simulink model "Turntable_close"  (R2017b)
settings: Solver=FixedStepAuto  StartTime=0.0  StopTime=10  FixedStep=0.0005  RelTol=1e-3
values from neighbouring files (symbols this model uses):
  bClose = 1    [sweep.m]
  bFt = 1    [sweep.m]
  bTf = 0    [sweep.m]
  fre = fre_array(i)    [sweep.m]
  J = 1.076    [sweep.m]
  Kps = 1.077250780790937e+02    (= 107.725078079)    [sweep.m]
  Kt = 24.812626200641272    (= 24.8126262006)    [sweep.m]
  Kv = 0.12    [sweep.m]
  L = 0.733240176511722    (= 0.733240176512)    [sweep.m]
  mag = 10 .^ (turntable_bode.mag / 20)    [sweep.m]    (also in test.m = ET205(1: 75, 1))
  r = 80.116666666666666667    (= 80.1166666667)    [sweep.m]
  t_off = 10    [sweep.m]
  Type = 1    [sweep.m]
settings Model: Creator=Vera  LastModifiedBy=surunbing
settings OptimizationCC: LifeSpan=inf
settings DebuggingCC: SFExecutionAtInitializationDiag=none
settings CodeAppCC: StateflowObjectComments=on

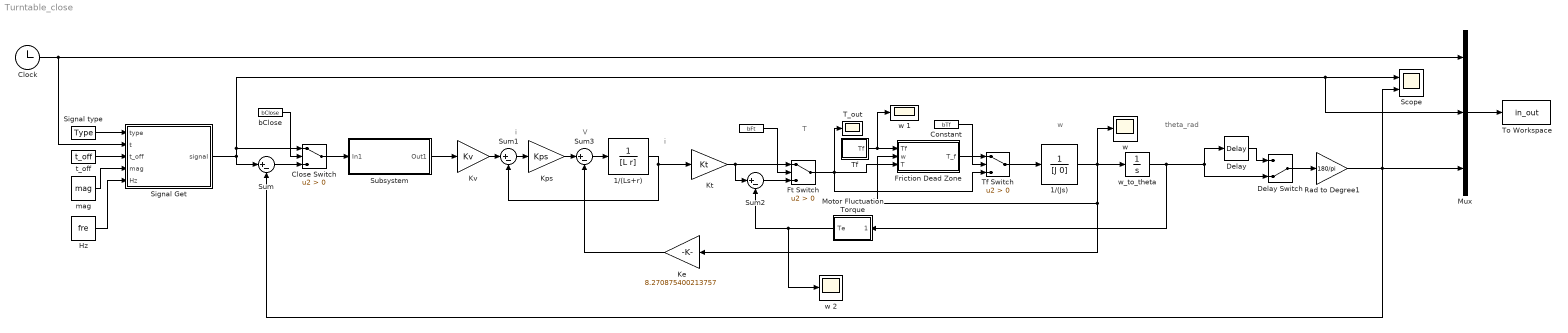
== system Turntable_close ==
  note: i
  note: w
  note: V
  note: i
  note: T
  note: theta_rad
  " " : Constant  Value=bFt
  " Delay Switch" : ManualSwitch  CurrentSetting=0
  " bClose" : Constant  Value=bClose
  1/(Js) : TransferFcn  Denominator=[J 0]
  1/(Ls+r) : TransferFcn  Denominator=[L r]
  Clock : Clock
  Close Switch : Switch  Criteria=u2 > Threshold
  Constant : Constant  Value=bTf
  Delay : TransportDelay  DelayTime=0.003763900000000
  Friction Dead Zone : MATLAB Function  TreatAsAtomicUnit=on
  Ft Switch : Switch  Criteria=u2 > Threshold
  Hz : Constant  Value=fre
  Ke : Gain  Gain=8.270875400213757
  Kps : Gain  Gain=Kps
  Kt : Gain  Gain=Kt
  Kv : Gain  Gain=Kv
  Motor Fluctuation Torque : Subsystem
  Mux : Mux  Inputs=3
  Rad to Degree1 : Gain  Gain=180/pi
  Scope : Scope  NumInputPorts=2
  Signal Get : MATLAB Function  TreatAsAtomicUnit=on
  Signal type : Constant  Value=Type
  Subsystem : Subsystem
  Sum{,1..3} (4 alike) : Sum  Inputs=|+-
  T_out : Scope
  Tf : Subsystem
  Tf Switch : Switch  Criteria=u2 > Threshold
  To Workspace : ToWorkspace  VariableName=in_out  SampleTime=-1
  mag : Constant  Value=mag
  t_off : Constant  Value=t_off
  "w " : Scope
  w 1 : Scope
  w 2 : Scope
  w_to_theta : Integrator
  wires:
  t_off/1 -> Signal Get/3(t_off)
  Clock/1 -> Mux/1, Signal Get/2(t)
  mag/1 -> Signal Get/4(mag)
  Hz/1 -> Signal Get/5(Hz)
  Kv/1 -> Sum1/1
  Motor Fluctuation Torque/1(Te) -> w 2/1, Sum2/2
  Tf/1(Tf) -> w 1/1, Friction Dead Zone/1(Tf)
  1/(Ls+r)/1 -> Sum1/2, Kt/1
  Rad to Degree1/1 -> Sum/2, Scope/2, Mux/3
  Sum3/1 -> 1/(Ls+r)/1
  Delay/1 -> " Delay Switch"/1
  w_to_theta/1 -> Delay/1, " Delay Switch"/2, Motor Fluctuation Torque/1(theta)
  " Delay Switch"/1 -> Rad to Degree1/1
  1/(Js)/1 -> "w "/1, w_to_theta/1, Friction Dead Zone/2(w), Ke/1
  Ke/1 -> Sum3/2
  Sum1/1 -> Kps/1
  Kt/1 -> Ft Switch/1, Sum2/1
  Kps/1 -> Sum3/1
  Mux/1 -> To Workspace/1
  Signal type/1 -> Signal Get/1(type)
  Subsystem/1(Out1) -> Kv/1
  Signal Get/1(signal) -> Sum/1, Close Switch/1, Mux/2, Scope/1
  Tf Switch/1 -> 1/(Js)/1
  Friction Dead Zone/1(T_f) -> Tf Switch/1
  Constant/1 -> Tf Switch/2
  Sum2/1 -> Ft Switch/3
  " "/1 -> Ft Switch/2
  Ft Switch/1 -> Friction Dead Zone/3(T), Tf Switch/3, T_out/1
  Close Switch/1 -> Subsystem/1(In1)
  Sum/1 -> Close Switch/3
  " bClose"/1 -> Close Switch/2

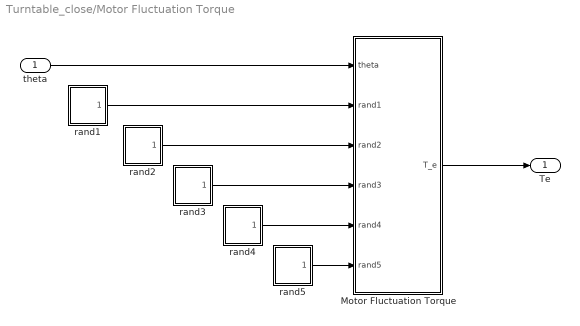
== system Turntable_close/Motor Fluctuation Torque ==
  theta : Inport
  Motor Fluctuation Torque : MATLAB Function  TreatAsAtomicUnit=on
  rand1 : Subsystem
  rand2 : Subsystem
  rand3 : Subsystem
  rand4 : Subsystem
  rand5 : Subsystem
  Te : Outport
  wires:
  theta/1 -> Motor Fluctuation Torque/1(theta)
  rand1/1(rand1) -> Motor Fluctuation Torque/2(rand1)
  rand2/1(rand2) -> Motor Fluctuation Torque/3(rand2)
  rand3/1(rand3) -> Motor Fluctuation Torque/4(rand3)
  rand4/1(rand4) -> Motor Fluctuation Torque/5(rand4)
  rand5/1(rand5) -> Motor Fluctuation Torque/6(rand5)
  Motor Fluctuation Torque/1(T_e) -> Te/1

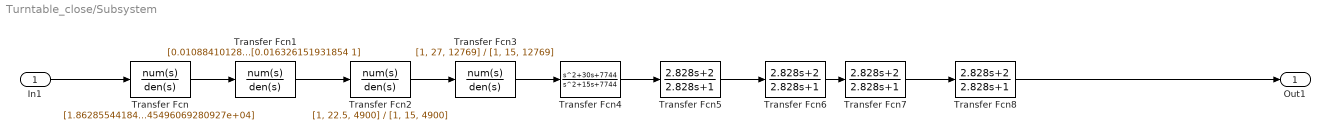
== system Turntable_close/Subsystem ==
  In1 : Inport
  Transfer Fcn : TransferFcn  Numerator=[1.862855441845868e+03, 4.791184320340544e+05, 4.845577407565945e+05]  Denominator=[0.069518879142540, 1.156462324547402e+02, 6.745496069280927e+04]
  Transfer Fcn1 : TransferFcn  Numerator=[0.010884101287903, 1] * 0.633290558182777  Denominator=[0.016326151931854 1]
  Transfer Fcn2 : TransferFcn  Numerator=[1, 22.5, 4900]  Denominator=[1, 15, 4900]
  Transfer Fcn3 : TransferFcn  Numerator=[1, 27, 12769]  Denominator=[1, 15, 12769]
  Transfer Fcn4 : TransferFcn  Numerator=[1, 30, 7744]  Denominator=[1, 15, 7744]
  Transfer Fcn{5..8} (4 alike) : TransferFcn  Numerator=[2.828, 2]  Denominator=[2.828, 1]
  Out1 : Outport
  wires:
  In1/1 -> Transfer Fcn/1
  Transfer Fcn/1 -> Transfer Fcn1/1
  Transfer Fcn1/1 -> Transfer Fcn2/1
  Transfer Fcn2/1 -> Transfer Fcn3/1
  Transfer Fcn3/1 -> Transfer Fcn4/1
  Transfer Fcn4/1 -> Transfer Fcn5/1
  Transfer Fcn5/1 -> Transfer Fcn6/1
  Transfer Fcn6/1 -> Transfer Fcn7/1
  Transfer Fcn7/1 -> Transfer Fcn8/1
  Transfer Fcn8/1 -> Out1/1

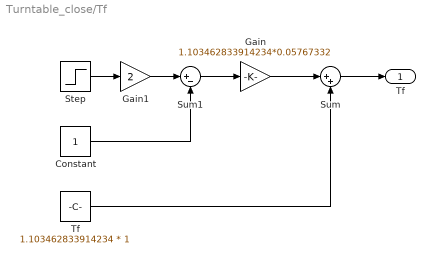
== system Turntable_close/Tf ==
  Constant : Constant
  Gain : Gain  Gain=1.103462833914234*0.05767332
  Gain1 : Gain  Gain=2
  Step : Step  Time=0  After=rand  SampleTime=0
  Sum : Sum  Inputs=|++
  Sum1 : Sum  Inputs=|+-
  "Tf " : Constant  Value=1.103462833914234 * 1  VectorParams1D=off
  Tf : Outport
  wires:
  Gain/1 -> Sum/1
  "Tf "/1 -> Sum/2
  Sum/1 -> Tf/1
  Step/1 -> Gain1/1
  Gain1/1 -> Sum1/1
  Constant/1 -> Sum1/2
  Sum1/1 -> Gain/1

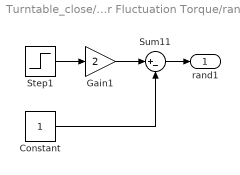
== system Turntable_close/Motor Fluctuation Torque/rand1 ==
  Constant : Constant
  Gain1 : Gain  Gain=2
  Step1 : Step  Time=0  After=rand  SampleTime=0
  Sum11 : Sum  Inputs=|+-
  rand1 : Outport
  wires:
  Step1/1 -> Gain1/1
  Gain1/1 -> Sum11/1
  Constant/1 -> Sum11/2
  Sum11/1 -> rand1/1

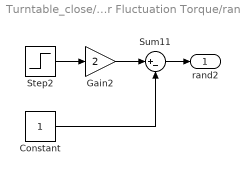
== system Turntable_close/Motor Fluctuation Torque/rand2 ==
  Constant : Constant
  Gain2 : Gain  Gain=2
  Step2 : Step  Time=0  After=rand  SampleTime=0
  Sum11 : Sum  Inputs=|+-
  rand2 : Outport
  wires:
  Step2/1 -> Gain2/1
  Gain2/1 -> Sum11/1
  Constant/1 -> Sum11/2
  Sum11/1 -> rand2/1

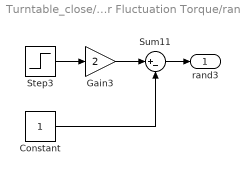
== system Turntable_close/Motor Fluctuation Torque/rand3 ==
  Constant : Constant
  Gain3 : Gain  Gain=2
  Step3 : Step  Time=0  After=rand  SampleTime=0
  Sum11 : Sum  Inputs=|+-
  rand3 : Outport
  wires:
  Sum11/1 -> rand3/1
  Constant/1 -> Sum11/2
  Gain3/1 -> Sum11/1
  Step3/1 -> Gain3/1

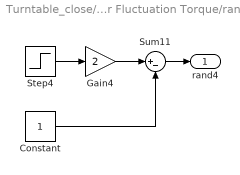
== system Turntable_close/Motor Fluctuation Torque/rand4 ==
  Constant : Constant
  Gain4 : Gain  Gain=2
  Step4 : Step  Time=0  After=rand  SampleTime=0
  Sum11 : Sum  Inputs=|+-
  rand4 : Outport
  wires:
  Step4/1 -> Gain4/1
  Gain4/1 -> Sum11/1
  Constant/1 -> Sum11/2
  Sum11/1 -> rand4/1

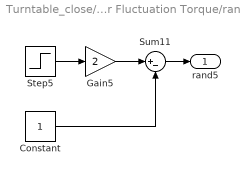
== system Turntable_close/Motor Fluctuation Torque/rand5 ==
  Constant : Constant
  Gain5 : Gain  Gain=2
  Step5 : Step  Time=0  After=rand  SampleTime=0
  Sum11 : Sum  Inputs=|+-
  rand5 : Outport
  wires:
  Sum11/1 -> rand5/1
  Constant/1 -> Sum11/2
  Gain5/1 -> Sum11/1
  Step5/1 -> Gain5/1

== matlab function Turntable_close/Signal Get ==
  data: type input; t input; t_off input; mag input; signal output; Hz input
function signal = fcn(type, t, t_off, mag, Hz)
signal = 0;
switch type
    case 1
        w = 2 * pi * Hz;
        if((t >= 0) && (t < 1))
            signal = t * mag * sin(w * t);
        elseif((t >= 1) && (t < t_off - 1))
            signal = mag * sin(w * t);
        elseif((t >= (t_off - 1)) && (t < t_off))
            signal = -mag * (t - t_off) * sin(w * t);
        else
            signal = 0;
        end
    case 2
        if t < 1
            signal = t * mag;
        elseif t >= 1 && t < (t_off - 1)
            signal = mag;
        elseif t >= (t_off - 1) && t < t_off
            signal = mag - (t_off - t) * mag;
        else
            signal = 0;
        end
        
end

== matlab function Turntable_close/Friction Dead Zone ==
  data: Tf input; w input; T input; T_f output
function T_f = fcn(Tf,w,T)
if w==0
    if abs(T)<abs(Tf)
        T_f = 0;
    else
        T_f=sign(T)*(abs(T)-Tf);
    end
elseif w*T<0
    T_f=sign(T)*(abs(T)+Tf);
else 
        if abs(T)<abs(Tf)
            T_f = -sign(w)*(Tf-abs(T));
        else
            T_f=sign(T)*(abs(T)-Tf);
        end

end
end

== matlab function Turntable_close/Motor Fluctuation Torque/Motor Fluctuation Torque ==
  data: T_e output; theta input; rand1 input; rand2 input; rand3 input; rand4 input; rand5 input
function T_e = fcn(theta,rand1,rand2,rand3,rand4,rand5)
T_p =0.432273269433135*(1+rand1*0.012015015613962)*cos(theta*7 +(48.13841636+0.050850865438431)*pi/180);
T_2p=0.035501355062786*(1+rand2*0.032198449030114)*cos(theta*14+(30.38979755+0.101746126073106)*pi/180);
T_4p=0.018930935537422*(1+rand3*0.028225982587057)*cos(theta*28+(285.7823597+0.203848223609672)*pi/180);
T_6p=0.012218243879728*(1+rand4*0.058230694793342)*cos(theta*42+(152.9148096+0.306666606518932)*pi/180);
T_45=0.009203318745614*(1+rand5*0.098213466988815)*cos(theta*45+(279.6898495+0.328827530537396)*pi/180);

T_e=1 * (T_p + T_2p + T_4p + T_6p + T_45);
end
